simulink library "powellsMethodMin_ul"  (R2018b)
settings: Solver=VariableStepAuto  StartTime=0.0  StopTime=10.0  RelTol=1e-3
values from neighbouring files (symbols this model uses):
  initialCoMPositionVec_cm = params.initCoMPosVec_cm.Value'    [snellsMin_ts.m]
  initialEulerAngles_rad = [0 0 0]'    [snellsMin_ts.m]
undefined symbols (not defined in the file or in its folder): params
settings Model: Creator=MAE-NCSUCORE  LastModifiedBy=MAE-NCSUCORE

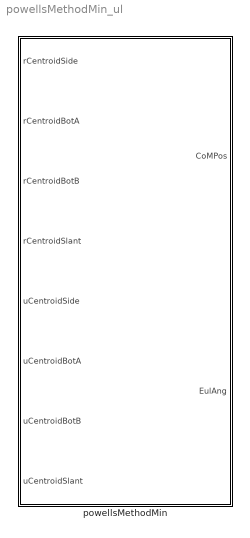
== system powellsMethodMin_ul ==
  powellsMethodMin : Subsystem  mask{sideDotPosVec_cm=params.sideDotPosVec_cm.Value, botADotPosVec_cm=params.botADotPosVec_cm.Value, botBDotPosVec_cm=params.botBDotPosVec_cm.Value, initialCoMPositionVec_cm=initialCoMPositionVec_cm, initialEulerAngles_rad=initialEulerAngles_rad}
      mask prompts: sideDotPosVec_cm "Side centroid position in body frame"; botADotPosVec_cm "Bottom A centroid position in body frame"; botBDotPosVec_cm "Bottom B centroid position in body frame"; initialCoMPositionVec_cm "Initial CoM Position Vector [cm]"; initialEulerAngles_rad "Initial Euler Angles [rad]"
      mask init:
      | powellsMethodMin_init;

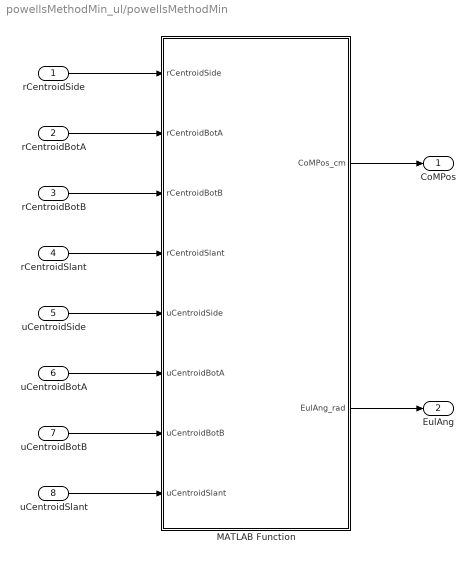
== system powellsMethodMin_ul/powellsMethodMin ==
  rCentroidSide : Inport
  rCentroidBotA : Inport  Port=2
  rCentroidBotB : Inport  Port=3
  rCentroidSlant : Inport  Port=4
  uCentroidSide : Inport  Port=5
  uCentroidBotA : Inport  Port=6
  uCentroidBotB : Inport  Port=7
  uCentroidSlant : Inport  Port=8
  MATLAB Function : MATLAB Function  TreatAsAtomicUnit=on
  CoMPos : Outport
  EulAng : Outport  Port=2
  wires:
  rCentroidBotA/1 -> MATLAB Function/2(rCentroidBotA)
  rCentroidBotB/1 -> MATLAB Function/3(rCentroidBotB)
  rCentroidSlant/1 -> MATLAB Function/4(rCentroidSlant)
  uCentroidBotB/1 -> MATLAB Function/7(uCentroidBotB)
  uCentroidSlant/1 -> MATLAB Function/8(uCentroidSlant)
  uCentroidBotA/1 -> MATLAB Function/6(uCentroidBotA)
  rCentroidSide/1 -> MATLAB Function/1(rCentroidSide)
  uCentroidSide/1 -> MATLAB Function/5(uCentroidSide)
  MATLAB Function/1(CoMPos_cm) -> CoMPos/1
  MATLAB Function/2(EulAng_rad) -> EulAng/1

== matlab function powellsMethodMin_ul/powellsMethodMin/MATLAB Function ==
  data: CoMPos_cm output; rCentroidSide input; rCentroidBotA input; rCentroidBotB input; rCentroidSlant input; uCentroidSide input; uCentroidBotA input; uCentroidBotB input; uCentroidSlant input; sideDotPosVec_cm parameter; EulAng_rad output; botADotPosVec_cm parameter; botBDotPosVec_cm parameter; initialEulerAngles_rad parameter; initialCoMPositionVec_cm parameter
function [CoMPos_cm,EulAng_rad] = powellsMethodMin(rCentroidSide,...
    rCentroidBotA,rCentroidBotB,rCentroidSlant,uCentroidSide,...
    uCentroidBotA,uCentroidBotB,uCentroidSlant,...
    sideDotPosVec_cm,botADotPosVec_cm,botBDotPosVec_cm,...
    initialEulerAngles_rad,initialCoMPositionVec_cm)

[CoMPos_cm,EulAng_rad] = powellsMethodMin(initialEulerAngles_rad,initialCoMPositionVec_cm,...
    rCentroidSide,rCentroidBotA,rCentroidBotB,rCentroidSlant,...
    uCentroidSide,uCentroidBotA,uCentroidBotB,uCentroidSlant,...
    sideDotPosVec_cm,botADotPosVec_cm,botBDotPosVec_cm);
